simulink model "quadcopter"  (R2023a)
settings: Solver=ode8  StartTime=0.0  StopTime=90  FixedStep=0.009  RelTol=1e-3
InitFcn:
  | addpath(fullfile(pwd, 'data'));  % Add 'data' folder relative to model location
  | run('param.m');
StopFcn:
  | addpath(fullfile(pwd, 'visualizer'));  % Add 'data' folder relative to model location
  | run('InteractiveFlightData.m');
undefined symbols (not defined in the file): attInit, b, d, g, Jm, Jx, Jy, Jz, Kp1H, Kp1Pitch, Kp1Roll, Kp1XY, Kp1Yaw, Kp2H, Kp2Pitch, Kp2Roll, Kp2XY, Kp2Yaw, Kt, Kth, l, m, motorSpinInit, omegaInit, posInit, Ra, u0, U1, velInit
libraries: SignalEditorBlockLib x1
settings Model: Creator=AlterraOnix  LastModifiedBy=AlterraOnix

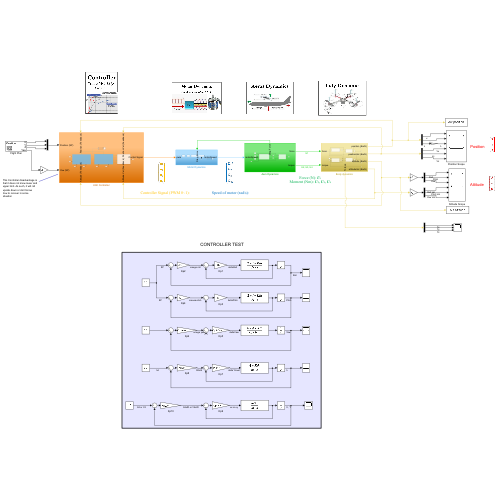
[thumbnail: Simulink's stored preview of the top-level diagram]
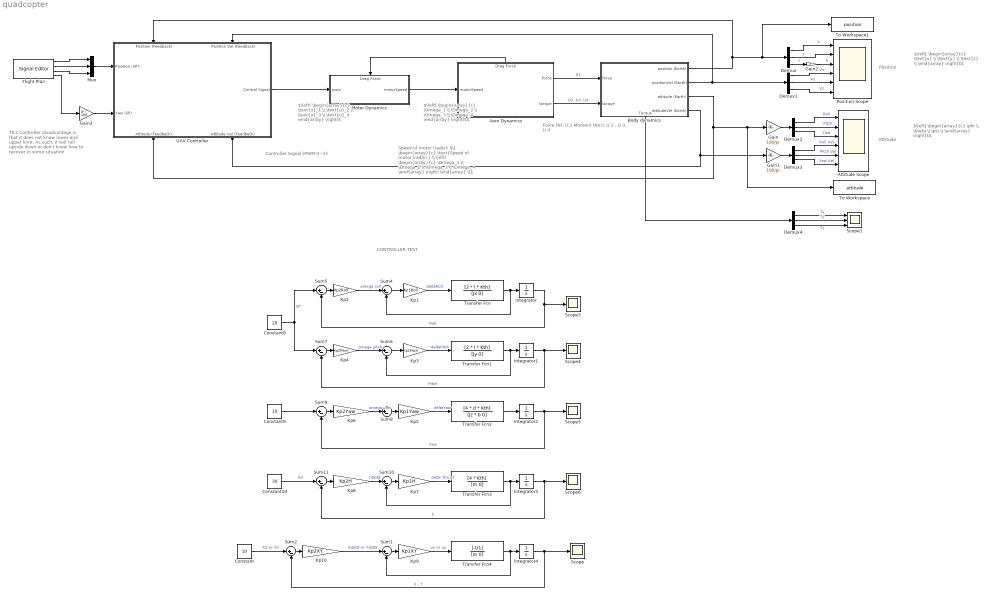
== system quadcopter ==
  note: This Controller disadvantage is that it does not know lower and upper limit. As such, it will roll upside down or don't know how to recover in some situation
  note: Controller Signal (PWM 0~1):
  note: Speed of motor (rad/s): $\[ \begin{array}{c} \text{Speed of motor (rad/s):} \\ \left( \begin{array}{c} \Omega_1 \\ \Omega_2 \\ \Omega_3 \\ \Omega_4 \end{array} \right) \end{array} \]$
  note: CONTROLLER TEST
  note: $\left( \begin{array}{c} \text{u}_1 \\ \text{u}_2 \\ \text{u}_3 \\ \text{u}_4 \end{array} \right)$
  note: $\left( \begin{array}{c} \Omega_1 \\ \Omega_2 \\ \Omega_3 \\ \Omega_4 \end{array} \right)$$
  note: $\left[ \begin{array}{c} \text{x} \\ \text{y} \\ \text{z} \\ \end{array} \right]$$
  note: Attitude
  note: Force (N): U 1
      | Moment (Nm): U 2 , U 3 , U 4
  note: $\left[ \begin{array}{c} \phi \\ \theta \\ \psi \\ \end{array} \right]$$
  note: Position
  Aero Dynamics : Subsystem
      settings: PortSchema="{\"entries\":[{\"content\":{\"sides\":[{\"content\":{\"connectorIds\":[\"In1\"]},\"type\":\"ConnectorPlacement.EquallySpacedRectSide\",\"uuid\":\"5da6d23f-8fa7-4c0d-a7a0-beca667c322f\"},{\"content\":{\"connectorIds\":[\"Out1\",\"Out2\"],\"side\":\"RIGHT\"},\"type\":\"ConnectorPlacement.EquallySpacedRectSide\",\"uuid\":\"114e7ba7-d132-465a-ab12-df00cea923bb\"},{\"content\":{\"connectorIds\":[\"Out3\"],\"side\":\"TOP\"},\"type\":\"ConnectorPlacement.EquallySpacedRectSide\",\"uuid\":\"e5217758-388b-4662-b4f7-0acce50e1924\"},{\"content\":{\"side\":\"BOTTOM\"},\"type\":\"ConnectorPlacement.EquallySpacedRectSide\",\"uuid\":\"6570f914-0b05-4701-b12c-fff372ec49f4\"}]},\"type\":\"ConnectorPlacement.EquallySpacedConnector\",\"uuid\":\"cad8bab3-1cdd-4308-8006-abeb193f8d84\"}],\"packageUris\":[\"http://schema.mathworks.com/mf0/Connector/R2020b\"],\"version\":\"1.0\"}"
  Attitude Scope : Scope  NumInputPorts=6
  Body dynamics : Subsystem
      settings: PortSchema="{\"entries\":[{\"content\":{\"sides\":[{\"content\":{\"connectorIds\":[\"In1\",\"In2\"]},\"type\":\"ConnectorPlacement.EquallySpacedRectSide\",\"uuid\":\"f237c637-46b2-45cc-89c7-502c3b4d3a82\"},{\"content\":{\"connectorIds\":[\"Out1\",\"Out2\",\"Out3\",\"Out4\"],\"side\":\"RIGHT\"},\"type\":\"ConnectorPlacement.EquallySpacedRectSide\",\"uuid\":\"40c9e1e3-93af-41ee-b851-152c56db6279\"},{\"content\":{\"side\":\"TOP\"},\"type\":\"ConnectorPlacement.EquallySpacedRectSide\",\"uuid\":\"88961279-dd7e-4791-8884-b5ffc6cf90cf\"},{\"content\":{\"connectorIds\":[\"Out5\"],\"side\":\"BOTTOM\"},\"type\":\"ConnectorPlacement.EquallySpacedRectSide\",\"uuid\":\"3396dfe3-4d1e-4c48-aaa0-4ba76fac5eff\"}]},\"type\":\"ConnectorPlacement.EquallySpacedConnector\",\"uuid\":\"743c7388-b4e3-439e-b61e-34a6bdced663\"}],\"packageUris\":[\"http://schema.mathworks.com/mf0/Connector/R2020b\"],\"version\":\"1.0\"}"
  Constant : Constant  Value=10
  Constant10 : Constant  Value=30
  Constant8 : Constant  Value=20
  Constant9 : Constant  Value=10
  Demux{,1..4} (5 alike) : Demux  Outputs=3
  Flight Plan : SignalEditorBlockLib/Signal Editor  FileName=flightPlan.mat  ActiveScenario=Position  ActiveSignal=X  IsBus=off  OutputBusObjectStr=Bus: BusObject  SampleTime=0  Interpolate=off  ZeroCross=off  OutputAfterFinalValue=Setting to zero  Unit=inherit  PreserveSignalName=on  ApplySigPropsToAllScenarios=on
  Gain : Gain  Gain=180/pi
  Gain1 : Gain  Gain=180/pi
  Gain2 : Gain  Gain=-1
  Gain3 : Gain  Gain=pi / 180
  Integrator{,1..4} (5 alike) : Integrator
  Kp1 : Gain  Gain=Kp1Roll
  Kp10 : Gain  Gain=Kp2XY
  Kp2 : Gain  Gain=Kp2Roll
  Kp3 : Gain  Gain=Kp1Pitch
  Kp4 : Gain  Gain=Kp2Pitch
  Kp5 : Gain  Gain=Kp1Yaw
  Kp6 : Gain  Gain=Kp2Yaw
  Kp7 : Gain  Gain=Kp1H
  Kp8 : Gain  Gain=Kp2H
  Kp9 : Gain  Gain=Kp1XY
  Motor Dynamics : Subsystem
      settings: PortSchema="{\"entries\":[{\"content\":{\"sides\":[{\"content\":{\"connectorIds\":[\"In1\"]},\"type\":\"ConnectorPlacement.EquallySpacedRectSide\",\"uuid\":\"1ed76e9c-5936-4080-821c-bad0eb24ae59\"},{\"content\":{\"connectorIds\":[\"Out1\"],\"side\":\"RIGHT\"},\"type\":\"ConnectorPlacement.EquallySpacedRectSide\",\"uuid\":\"bcce61fc-9c46-4acb-991d-be4c01e36c5c\"},{\"content\":{\"connectorIds\":[\"In2\"],\"side\":\"TOP\"},\"type\":\"ConnectorPlacement.EquallySpacedRectSide\",\"uuid\":\"b76f1f95-13d4-401e-9c02-e7da8ef90a20\"},{\"content\":{\"side\":\"BOTTOM\"},\"type\":\"ConnectorPlacement.EquallySpacedRectSide\",\"uuid\":\"72a5d901-ef88-4b44-b58a-8f83b182bcfd\"}]},\"type\":\"ConnectorPlacement.EquallySpacedConnector\",\"uuid\":\"e2e8c0d7-4140-446e-9fb7-4366562bc7fa\"}],\"packageUris\":[\"http://schema.mathworks.com/mf0/Connector/R2020b\"],\"version\":\"1.0\"}"
  Mux : Mux  Inputs=3
  Position Scope : Scope  NumInputPorts=6
  Scope{,3..6} (5 alike) : Scope
  Scope1 : Scope  NumInputPorts=3
  Sum{1..2,4..11} (10 alike) : Sum  Inputs=|+-
  To Workspace : ToWorkspace  VariableName=attitude  SaveFormat=Timeseries  SampleTime=-1
  To Workspace1 : ToWorkspace  VariableName=position  SaveFormat=Timeseries  SampleTime=-1
  Transfer Fcn : TransferFcn  Numerator=[2 * l * Kth]  Denominator=[Jx 0]
  Transfer Fcn1 : TransferFcn  Numerator=[2 * l * Kth]  Denominator=[Jy 0]
  Transfer Fcn2 : TransferFcn  Numerator=[4 * d * Kth]  Denominator=[Jz * b 0]
  Transfer Fcn3 : TransferFcn  Numerator=[4 * Kth]  Denominator=[m 0]
  Transfer Fcn4 : TransferFcn  Numerator=[-U1]  Denominator=[m 0]
  UAV Controller : Subsystem
      settings: PortSchema="{\"entries\":[{\"content\":{\"sides\":[{\"content\":{\"connectorIds\":[\"In1\",\"In2\"]},\"type\":\"ConnectorPlacement.EquallySpacedRectSide\",\"uuid\":\"50802edf-a040-4c28-b591-d88e611188de\"},{\"content\":{\"connectorIds\":[\"Out1\"],\"side\":\"RIGHT\"},\"type\":\"ConnectorPlacement.EquallySpacedRectSide\",\"uuid\":\"dce66916-8d71-4fa6-a653-99da5dcfcd3d\"},{\"content\":{\"connectorIds\":[\"In3\",\"In4\"],\"side\":\"TOP\"},\"type\":\"ConnectorPlacement.EquallySpacedRectSide\",\"uuid\":\"d9b7a688-6099-435e-b59a-2f38cb1d0a01\"},{\"content\":{\"connectorIds\":[\"In5\",\"In6\"],\"side\":\"BOTTOM\"},\"type\":\"ConnectorPlacement.EquallySpacedRectSide\",\"uuid\":\"81b63a5f-7537-41dc-8937-f7595f7d4ca8\"}]},\"type\":\"ConnectorPlacement.EquallySpacedConnector\",\"uuid\":\"c3f81b6a-8709-448a-9549-898422283d5d\"}],\"packageUris\":[\"http://schema.mathworks.com/mf0/Connector/R2020b\"],\"version\":\"1.0\"}"
  wires:
  Transfer Fcn/1 -> Sum4/2, Integrator/1
  Kp1/1 -> Transfer Fcn/1  "deltaRoll"
  Sum4/1 -> Kp1/1
  Sum5/1 -> Kp2/1
  Kp2/1 -> Sum4/1  "omega roll"
  Integrator/1 -> Sum5/2, Scope3/1  "Roll"
  Integrator1/1 -> Scope4/1, Sum7/2  "Pitch"
  Sum7/1 -> Kp4/1
  Transfer Fcn1/1 -> Sum6/2, Integrator1/1
  Kp3/1 -> Transfer Fcn1/1  "deltaPitch"
  Sum6/1 -> Kp3/1
  Kp4/1 -> Sum6/1  "omega pitch"
  Kp6/1 -> Sum8/1  "omega yaw"
  Sum8/1 -> Kp5/1
  Integrator2/1 -> Scope5/1, Sum9/2  "Yaw"
  Kp5/1 -> Transfer Fcn2/1  "deltaYaw"
  Constant8/1 -> Sum7/1, Sum5/1  "SP"
  Sum9/1 -> Kp6/1
  Constant9/1 -> Sum9/1
  Transfer Fcn3/1 -> Sum10/2, Integrator3/1
  Integrator3/1 -> Scope6/1, Sum11/2  "h"
  Kp8/1 -> Sum10/1  "hDotd"
  Sum11/1 -> Kp8/1
  Kp7/1 -> Transfer Fcn3/1  "delta' thrust"
  Sum10/1 -> Kp7/1
  Constant10/1 -> Sum11/1  "hd"
  Constant/1 -> Sum2/1  "Xd or Yd"
  Kp9/1 -> Transfer Fcn4/1  "ux or uy"
  Sum2/1 -> Kp10/1
  Kp10/1 -> Sum1/1  "XdotD or YdotD"
  Transfer Fcn4/1 -> Sum1/2, Integrator4/1
  Sum1/1 -> Kp9/1
  Integrator4/1 -> Sum2/2, Scope/1  "X , Y"
  Mux/1 -> UAV Controller/1(Position (SP))
  Demux1/3 -> Position Scope/6  "Vz"
  Demux1/2 -> Position Scope/5  "Vy"
  Demux1/1 -> Position Scope/4  "Vx"
  Demux/2 -> Position Scope/2  "y"
  Demux/1 -> Position Scope/1  "x"
  Gain/1 -> Demux2/1
  Demux2/1 -> Attitude Scope/1  "Roll"
  Demux2/2 -> Attitude Scope/2  "Pitch"
  Demux2/3 -> Attitude Scope/3  "Yaw"
  Gain1/1 -> Demux3/1
  Demux3/1 -> Attitude Scope/4  "Roll Vel"
  Demux3/2 -> Attitude Scope/5  "Pitch Vel"
  Demux3/3 -> Attitude Scope/6  "Yaw Vel"
  Gain2/1 -> Position Scope/3  "h"
  Demux/3 -> Gain2/1  "z"
  UAV Controller/1(Control Signal) -> Motor Dynamics/1(pwm)
  Aero Dynamics/1(force) -> Body dynamics/1(force)  "U1"
  Aero Dynamics/3(Drag Force) -> Motor Dynamics/2(Drag Force)
  Motor Dynamics/1(motorSpeed) -> Aero Dynamics/1(motorSpeed)
  Aero Dynamics/2(torque) -> Body dynamics/2(torque)  "U2, U3, U4"
  Body dynamics/4(attitudeVel (Earth)) -> Gain1/1, UAV Controller/6(Attitude Vel (Feedback))
  Body dynamics/3(attitude (Earth)) -> To Workspace/1, Gain/1, UAV Controller/5(Attitude (Feedback))
  Body dynamics/2(positionVel (Earth)) -> Demux1/1, UAV Controller/4(Position Vel (Feedback))
  Body dynamics/1(position (Earth)) -> UAV Controller/3(Position (Feedback)), To Workspace1/1, Demux/1
  Gain3/1 -> UAV Controller/2(Yaw (SP))
  Body dynamics/5(Torque) -> Demux4/1
  Demux4/3 -> Scope1/3  "Tz"
  Demux4/2 -> Scope1/2  "Ty"
  Demux4/1 -> Scope1/1  "Tx"
  Flight Plan/1 -> Mux/1
  Flight Plan/2 -> Mux/2
  Flight Plan/3 -> Mux/3
  Flight Plan/4 -> Gain3/1
  Transfer Fcn2/1 -> Integrator2/1

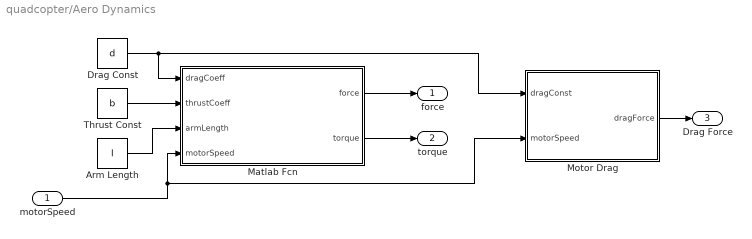
== system quadcopter/Aero Dynamics ==
  motorSpeed : Inport
  Arm Length : Constant  Value=l
  Drag Const : Constant  Value=d
  Matlab Fcn : MATLAB Function  TreatAsAtomicUnit=on
  Motor Drag : MATLAB Function  TreatAsAtomicUnit=on
  Thrust Const : Constant  Value=b
  force : Outport
  torque : Outport  Port=2
  Drag Force : Outport  Port=3
  wires:
  Drag Const/1 -> Motor Drag/1(dragConst), Matlab Fcn/1(dragCoeff)
  Arm Length/1 -> Matlab Fcn/3(armLength)
  Thrust Const/1 -> Matlab Fcn/2(thrustCoeff)
  motorSpeed/1 -> Motor Drag/2(motorSpeed), Matlab Fcn/4(motorSpeed)
  Matlab Fcn/1(force) -> force/1
  Motor Drag/1(dragForce) -> Drag Force/1
  Matlab Fcn/2(torque) -> torque/1

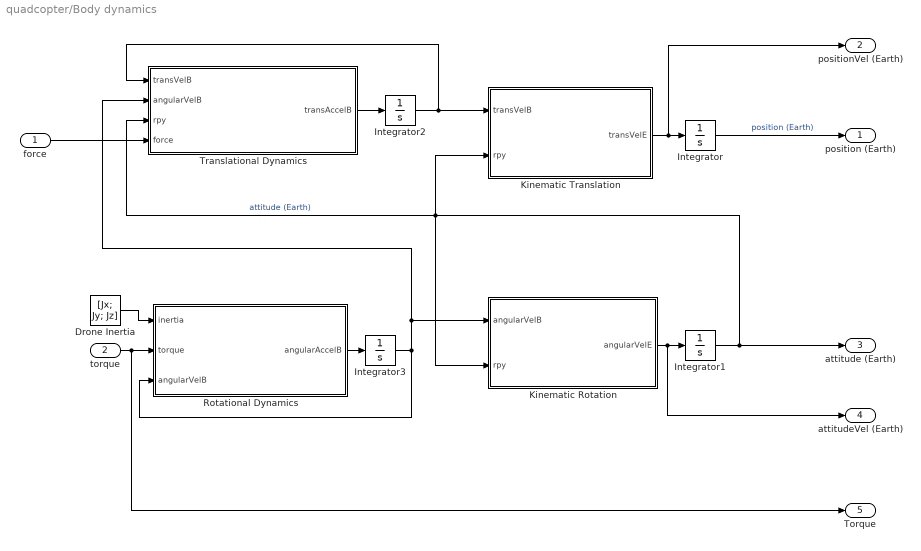
== system quadcopter/Body dynamics ==
  force : Inport
  torque : Inport  Port=2
  Drone Inertia : Constant  Value=[Jx; Jy; Jz]
  Integrator : Integrator  InitialCondition=posInit
  Integrator1 : Integrator  InitialCondition=attInit
  Integrator2 : Integrator  InitialCondition=velInit
  Integrator3 : Integrator  InitialCondition=omegaInit
  Kinematic Rotation : MATLAB Function  TreatAsAtomicUnit=on
  Kinematic Translation : MATLAB Function  TreatAsAtomicUnit=on
  Rotational Dynamics : MATLAB Function  TreatAsAtomicUnit=on
  Translational Dynamics : Subsystem
  position (Earth) : Outport
  positionVel (Earth) : Outport  Port=2
  attitude (Earth) : Outport  Port=3
  attitudeVel (Earth) : Outport  Port=4
  Torque : Outport  Port=5
  wires:
  Kinematic Rotation/1(angularVelE) -> attitudeVel (Earth)/1, Integrator1/1
  Drone Inertia/1 -> Rotational Dynamics/1(inertia)
  Translational Dynamics/1(transAccelB) -> Integrator2/1
  Kinematic Translation/1(transVelE) -> positionVel (Earth)/1, Integrator/1
  Rotational Dynamics/1(angularAccelB) -> Integrator3/1
  Integrator2/1 -> Translational Dynamics/1(transVelB), Kinematic Translation/1(transVelB)
  Integrator1/1 -> Translational Dynamics/3(rpy), Kinematic Rotation/2(rpy), Kinematic Translation/2(rpy), attitude (Earth)/1  "attitude (Earth)"
  Integrator/1 -> position (Earth)/1  "position (Earth)"
  Integrator3/1 -> Rotational Dynamics/3(angularVelB), Translational Dynamics/2(angularVelB), Kinematic Rotation/1(angularVelB)
  torque/1 -> Torque/1, Rotational Dynamics/2(torque)
  force/1 -> Translational Dynamics/4(force)

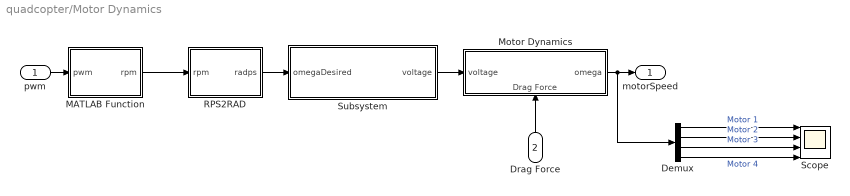
== system quadcopter/Motor Dynamics ==
  pwm : Inport
  Drag Force : Inport  Port=2
  Demux : Demux
  MATLAB Function : MATLAB Function  TreatAsAtomicUnit=on
  Motor Dynamics : Subsystem
      settings: PortSchema="{\"entries\":[{\"content\":{\"sides\":[{\"content\":{\"connectorIds\":[\"In1\"]},\"type\":\"ConnectorPlacement.EquallySpacedRectSide\",\"uuid\":\"c533e7cd-ee38-4db5-be38-3827405b94e5\"},{\"content\":{\"connectorIds\":[\"Out1\"],\"side\":\"RIGHT\"},\"type\":\"ConnectorPlacement.EquallySpacedRectSide\",\"uuid\":\"e10529f3-e7e6-435f-ba64-638186187bc4\"},{\"content\":{\"side\":\"TOP\"},\"type\":\"ConnectorPlacement.EquallySpacedRectSide\",\"uuid\":\"af8a99ba-dd5a-4918-9e60-3f38c4f7af03\"},{\"content\":{\"connectorIds\":[\"In2\"],\"side\":\"BOTTOM\"},\"type\":\"ConnectorPlacement.EquallySpacedRectSide\",\"uuid\":\"cc26d8fe-22a0-44bc-9eba-a7f7a779408e\"}]},\"type\":\"ConnectorPlacement.EquallySpacedConnector\",\"uuid\":\"51d375ef-3caf-4fe1-845a-afb7267c381d\"}],\"packageUris\":[\"http://schema.mathworks.com/mf0/Connector/R2020b\"],\"version\":\"1.0\"}"
  RPS2RAD : MATLAB Function  TreatAsAtomicUnit=on
  Scope : Scope  NumInputPorts=4
  Subsystem : Subsystem
  motorSpeed : Outport
  wires:
  Subsystem/1(voltage) -> Motor Dynamics/1(voltage)
  Motor Dynamics/1(omega) -> Demux/1, motorSpeed/1
  Drag Force/1 -> Motor Dynamics/2(Drag Force)
  MATLAB Function/1(rpm) -> RPS2RAD/1(rpm)
  pwm/1 -> MATLAB Function/1(pwm)
  RPS2RAD/1(radps) -> Subsystem/1(omegaDesired)
  Demux/1 -> Scope/1  "Motor 1"
  Demux/2 -> Scope/2  "Motor 2"
  Demux/3 -> Scope/3  "Motor 3"
  Demux/4 -> Scope/4  "Motor 4"

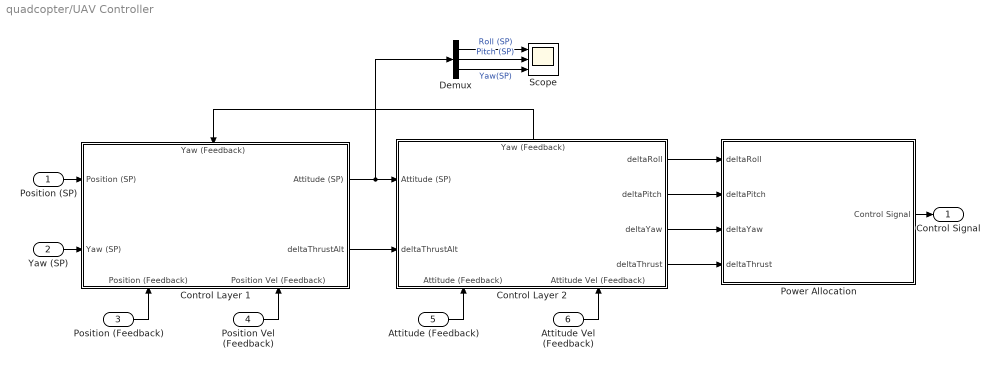
== system quadcopter/UAV Controller ==
  Position (SP) : Inport
  Yaw (SP) : Inport  Port=2
  Position (Feedback) : Inport  Port=3
  Position Vel (Feedback) : Inport  Port=4
  Attitude (Feedback) : Inport  Port=5
  Attitude Vel (Feedback) : Inport  Port=6
  Control Layer 1 : Subsystem
      settings: PortSchema="{\"entries\":[{\"content\":{\"sides\":[{\"content\":{\"connectorIds\":[\"In1\",\"In2\"]},\"type\":\"ConnectorPlacement.EquallySpacedRectSide\",\"uuid\":\"e1a47314-e725-4ad2-912f-1a38871ee891\"},{\"content\":{\"connectorIds\":[\"Out1\",\"Out2\"],\"side\":\"RIGHT\"},\"type\":\"ConnectorPlacement.EquallySpacedRectSide\",\"uuid\":\"53b24631-b87e-42e7-944b-57bbc6991867\"},{\"content\":{\"connectorIds\":[\"In3\"],\"side\":\"TOP\"},\"type\":\"ConnectorPlacement.EquallySpacedRectSide\",\"uuid\":\"7fd7a42b-f6aa-4761-a0eb-10b11e6a4f43\"},{\"content\":{\"connectorIds\":[\"In4\",\"In5\"],\"side\":\"BOTTOM\"},\"type\":\"ConnectorPlacement.EquallySpacedRectSide\",\"uuid\":\"80c3e12e-deab-4463-bb3e-5443ff9a6220\"}]},\"type\":\"ConnectorPlacement.EquallySpacedConnector\",\"uuid\":\"e52dd722-c82f-474b-bf17-6318b1f157b3\"}],\"packageUris\":[\"http://schema.mathworks.com/mf0/Connector/R2020b\"],\"version\":\"1.0\"}"
  Control Layer 2 : Subsystem
      settings: PortSchema="{\"entries\":[{\"content\":{\"sides\":[{\"content\":{\"connectorIds\":[\"In1\",\"In2\"]},\"type\":\"ConnectorPlacement.EquallySpacedRectSide\",\"uuid\":\"ca8a29f1-d2a3-473a-82ed-9fe12abcceea\"},{\"content\":{\"connectorIds\":[\"Out1\",\"Out2\",\"Out3\",\"Out4\"],\"side\":\"RIGHT\"},\"type\":\"ConnectorPlacement.EquallySpacedRectSide\",\"uuid\":\"e4ee1971-4b00-410f-bb76-76195639c31e\"},{\"content\":{\"connectorIds\":[\"Out5\"],\"side\":\"TOP\"},\"type\":\"ConnectorPlacement.EquallySpacedRectSide\",\"uuid\":\"3619c6cc-5c83-4adf-914e-d0bdc3e41505\"},{\"content\":{\"connectorIds\":[\"In3\",\"In4\"],\"side\":\"BOTTOM\"},\"type\":\"ConnectorPlacement.EquallySpacedRectSide\",\"uuid\":\"42efcdc0-00f6-4a08-9fda-d07be9cd5595\"}]},\"type\":\"ConnectorPlacement.EquallySpacedConnector\",\"uuid\":\"bb536f40-a213-48a0-8d9b-f4246912eccc\"}],\"packageUris\":[\"http://schema.mathworks.com/mf0/Connector/R2020b\"],\"version\":\"1.0\"}"
  Demux : Demux  Outputs=3
  Power Allocation : Subsystem
  Scope : Scope  NumInputPorts=3
  Control Signal : Outport
  wires:
  Attitude (Feedback)/1 -> Control Layer 2/3(Attitude (Feedback))
  Control Layer 2/4(deltaThrust) -> Power Allocation/4(deltaThrust)
  Control Layer 2/2(deltaPitch) -> Power Allocation/2(deltaPitch)
  Control Layer 1/1(Attitude (SP)) -> Demux/1, Control Layer 2/1(Attitude (SP))
  Control Layer 2/5(Yaw (Feedback)) -> Control Layer 1/3(Yaw (Feedback))
  Control Layer 2/3(deltaYaw) -> Power Allocation/3(deltaYaw)
  Control Layer 2/1(deltaRoll) -> Power Allocation/1(deltaRoll)
  Control Layer 1/2(deltaThrustAlt) -> Control Layer 2/2(deltaThrustAlt)
  Position (SP)/1 -> Control Layer 1/1(Position (SP))
  Attitude Vel (Feedback)/1 -> Control Layer 2/4(Attitude Vel (Feedback))
  Yaw (SP)/1 -> Control Layer 1/2(Yaw (SP))
  Position (Feedback)/1 -> Control Layer 1/4(Position (Feedback))
  Power Allocation/1(Control Signal) -> Control Signal/1
  Position Vel (Feedback)/1 -> Control Layer 1/5(Position Vel (Feedback))
  Demux/1 -> Scope/1  "Roll (SP)"
  Demux/2 -> Scope/2  "Pitch (SP)"
  Demux/3 -> Scope/3  "Yaw(SP)"

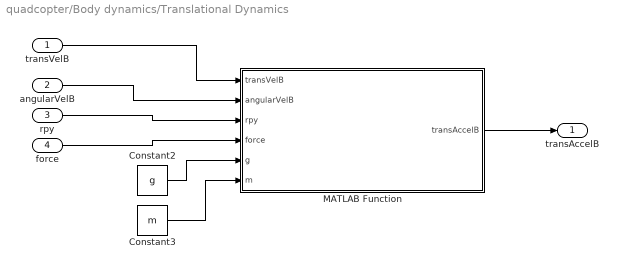
== system quadcopter/Body dynamics/Translational Dynamics ==
  transVelB : Inport
  angularVelB : Inport  Port=2
  rpy : Inport  Port=3
  force : Inport  Port=4
  Constant2 : Constant  Value=g
  Constant3 : Constant  Value=m
  MATLAB Function : MATLAB Function  TreatAsAtomicUnit=on
  transAccelB : Outport
  wires:
  rpy/1 -> MATLAB Function/3(rpy)
  transVelB/1 -> MATLAB Function/1(transVelB)
  Constant2/1 -> MATLAB Function/5(g)
  force/1 -> MATLAB Function/4(force)
  Constant3/1 -> MATLAB Function/6(m)
  angularVelB/1 -> MATLAB Function/2(angularVelB)
  MATLAB Function/1(transAccelB) -> transAccelB/1

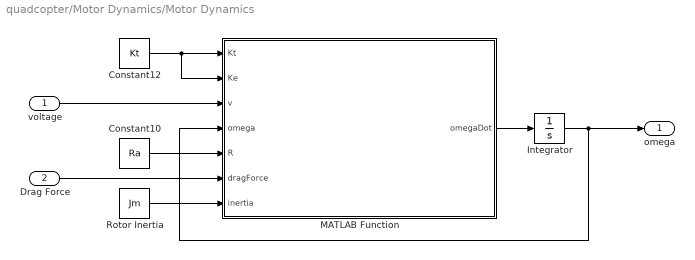
== system quadcopter/Motor Dynamics/Motor Dynamics ==
  voltage : Inport
  Drag Force : Inport  Port=2
  Constant10 : Constant  Value=Ra
  Constant12 : Constant  Value=Kt
  Integrator : Integrator  InitialCondition=motorSpinInit
  MATLAB Function : MATLAB Function  TreatAsAtomicUnit=on
  Rotor Inertia : Constant  Value=Jm
  omega : Outport
  wires:
  Constant12/1 -> MATLAB Function/1(Kt), MATLAB Function/2(Ke)
  voltage/1 -> MATLAB Function/3(v)
  Integrator/1 -> omega/1, MATLAB Function/4(omega)
  MATLAB Function/1(omegaDot) -> Integrator/1
  Constant10/1 -> MATLAB Function/5(R)
  Rotor Inertia/1 -> MATLAB Function/7(inertia)
  Drag Force/1 -> MATLAB Function/6(dragForce)

== system quadcopter/Motor Dynamics/Subsystem ==
  omegaDesired : Inport
  Constant13 : Constant  Value=Ra
  Constant14 : Constant  Value=d
  Constant15 : Constant  Value=Kt
  MATLAB Function : MATLAB Function  TreatAsAtomicUnit=on
  voltage : Outport
  wires:
  Constant13/1 -> MATLAB Function/5(Ra)
  MATLAB Function/1(voltage) -> voltage/1
  omegaDesired/1 -> MATLAB Function/1(omegaDesired)
  Constant15/1 -> MATLAB Function/2(Ke), MATLAB Function/3(Kt)
  Constant14/1 -> MATLAB Function/4(d)

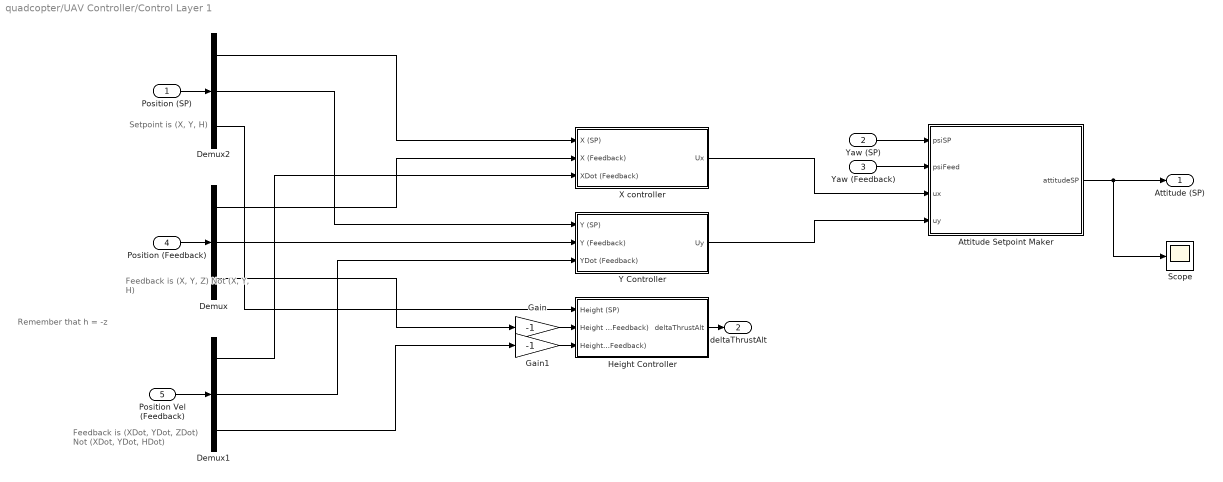
== system quadcopter/UAV Controller/Control Layer 1 ==
  note: Feedback is (X, Y, Z)
      | Not (X, Y, H)
  note: Remember that h = -z
  note: Feedback is (XDot, YDot, ZDot)
      | Not (XDot, YDot, HDot)
  note: Setpoint is (X, Y, H)
  Position (SP) : Inport
  Yaw (SP) : Inport  Port=2
  Yaw (Feedback) : Inport  Port=3
  Position (Feedback) : Inport  Port=4
  Position Vel (Feedback) : Inport  Port=5
  Attitude Setpoint Maker : MATLAB Function  TreatAsAtomicUnit=on
  Demux : Demux  Outputs=3
  Demux1 : Demux  Outputs=3
  Demux2 : Demux  Outputs=3
  Gain : Gain  Gain=-1
  Gain1 : Gain  Gain=-1
  Height Controller : Subsystem
  Scope : Scope
  X controller : Subsystem
  Y Controller : Subsystem
  Attitude (SP) : Outport
  deltaThrustAlt : Outport  Port=2
  wires:
  Height Controller/1(deltaThrustAlt) -> deltaThrustAlt/1
  Position (Feedback)/1 -> Demux/1
  Demux/1 -> X controller/2(X (Feedback))
  Demux/2 -> Y Controller/2(Y (Feedback))
  Gain/1 -> Height Controller/2(Height (Feedback))
  Demux/3 -> Gain/1
  Position Vel (Feedback)/1 -> Demux1/1
  Gain1/1 -> Height Controller/3(HeightDot (Feedback))
  Demux1/3 -> Gain1/1
  Demux1/2 -> Y Controller/3(YDot (Feedback))
  Demux1/1 -> X controller/3(XDot (Feedback))
  Position (SP)/1 -> Demux2/1
  Demux2/1 -> X controller/1(X (SP))
  Demux2/2 -> Y Controller/1(Y (SP))
  Demux2/3 -> Height Controller/1(Height (SP))
  Attitude Setpoint Maker/1(attitudeSP) -> Scope/1, Attitude (SP)/1
  Yaw (SP)/1 -> Attitude Setpoint Maker/1(psiSP)
  X controller/1(Ux) -> Attitude Setpoint Maker/3(ux)
  Y Controller/1(Uy) -> Attitude Setpoint Maker/4(uy)
  Yaw (Feedback)/1 -> Attitude Setpoint Maker/2(psiFeed)

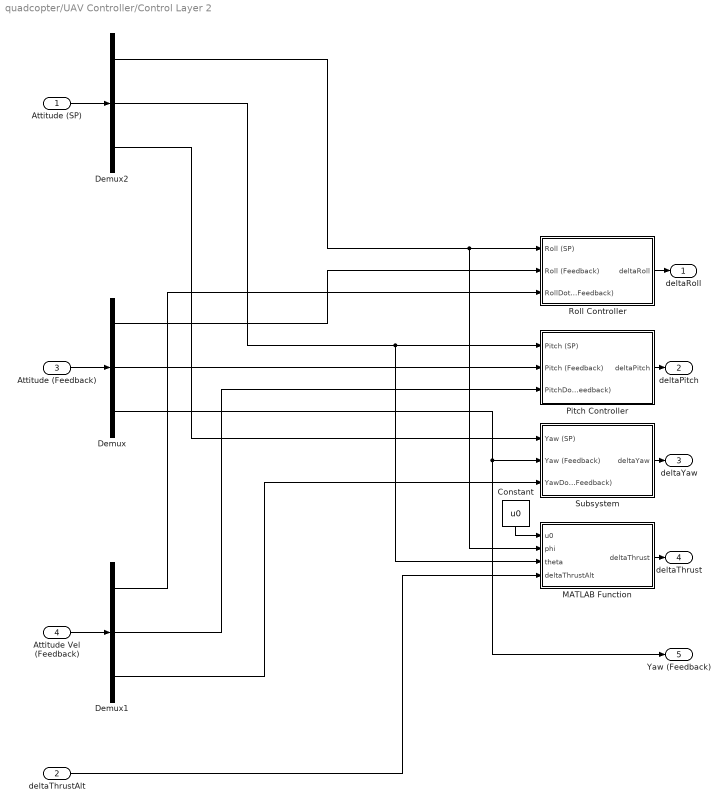
== system quadcopter/UAV Controller/Control Layer 2 ==
  Attitude (SP) : Inport
  deltaThrustAlt : Inport  Port=2
  Attitude (Feedback) : Inport  Port=3
  Attitude Vel (Feedback) : Inport  Port=4
  Constant : Constant  Value=u0
  Demux : Demux  Outputs=3
  Demux1 : Demux  Outputs=3
  Demux2 : Demux  Outputs=3
  MATLAB Function : MATLAB Function  TreatAsAtomicUnit=on
  Pitch Controller : Subsystem
  Roll Controller : Subsystem
  Subsystem : Subsystem
  deltaRoll : Outport
  deltaPitch : Outport  Port=2
  deltaYaw : Outport  Port=3
  deltaThrust : Outport  Port=4
  Yaw (Feedback) : Outport  Port=5
  wires:
  Demux/1 -> Roll Controller/2(Roll (Feedback))
  Roll Controller/1(deltaRoll) -> deltaRoll/1
  Demux1/1 -> Roll Controller/3(RollDot (Feedback))
  Subsystem/1(deltaYaw) -> deltaYaw/1
  Demux/3 -> Yaw (Feedback)/1, Subsystem/2(Yaw (Feedback))
  Demux1/3 -> Subsystem/3(YawDot (Feedback))
  Demux1/2 -> Pitch Controller/3(PitchDot (Feedback))
  Demux/2 -> Pitch Controller/2(Pitch (Feedback))
  Pitch Controller/1(deltaPitch) -> deltaPitch/1
  Attitude (Feedback)/1 -> Demux/1
  Attitude Vel (Feedback)/1 -> Demux1/1
  Attitude (SP)/1 -> Demux2/1
  Demux2/1 -> MATLAB Function/2(phi), Roll Controller/1(Roll (SP))
  Demux2/2 -> MATLAB Function/3(theta), Pitch Controller/1(Pitch (SP))
  Demux2/3 -> Subsystem/1(Yaw (SP))
  deltaThrustAlt/1 -> MATLAB Function/4(deltaThrustAlt)
  MATLAB Function/1(deltaThrust) -> deltaThrust/1
  Constant/1 -> MATLAB Function/1(u0)

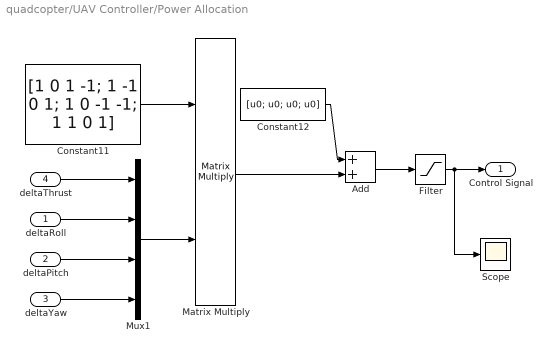
== system quadcopter/UAV Controller/Power Allocation ==
  deltaRoll : Inport
  deltaPitch : Inport  Port=2
  deltaYaw : Inport  Port=3
  deltaThrust : Inport  Port=4
  Add : Sum
  Constant11 : Constant  Value=[1 0 1 -1; 1 -1 0 1; 1 0 -1 -1; 1 1 0 1]
  Constant12 : Constant  Value=[u0; u0; u0; u0]
  Filter : Saturate  UpperLimit=1  LowerLimit=0
  Matrix Multiply : Product  Multiplication=Matrix(*)
  Mux1 : Mux
  Scope : Scope
  Control Signal : Outport
  wires:
  Mux1/1 -> Matrix Multiply/2
  Constant11/1 -> Matrix Multiply/1
  Constant12/1 -> Add/1
  Matrix Multiply/1 -> Add/2
  Filter/1 -> Scope/1, Control Signal/1
  Add/1 -> Filter/1
  deltaPitch/1 -> Mux1/3
  deltaYaw/1 -> Mux1/4
  deltaRoll/1 -> Mux1/2
  deltaThrust/1 -> Mux1/1

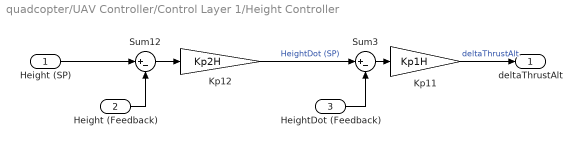
== system quadcopter/UAV Controller/Control Layer 1/Height Controller ==
  Height (SP) : Inport
  Height (Feedback) : Inport  Port=2
  HeightDot (Feedback) : Inport  Port=3
  Kp11 : Gain  Gain=Kp1H
  Kp12 : Gain  Gain=Kp2H
  Sum12 : Sum  Inputs=|+-
  Sum3 : Sum  Inputs=|+-
  deltaThrustAlt : Outport
  wires:
  Kp11/1 -> deltaThrustAlt/1  "deltaThrustAlt"
  Sum3/1 -> Kp11/1
  Sum12/1 -> Kp12/1
  Height (Feedback)/1 -> Sum12/2
  Kp12/1 -> Sum3/1  "HeightDot (SP)"
  Height (SP)/1 -> Sum12/1
  HeightDot (Feedback)/1 -> Sum3/2

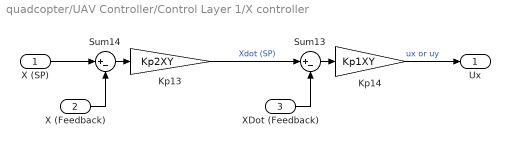
== system quadcopter/UAV Controller/Control Layer 1/X controller ==
  X (SP) : Inport
  X (Feedback) : Inport  Port=2
  XDot (Feedback) : Inport  Port=3
  Kp13 : Gain  Gain=Kp2XY
  Kp14 : Gain  Gain=Kp1XY
  Sum13 : Sum  Inputs=|+-
  Sum14 : Sum  Inputs=|+-
  Ux : Outport
  wires:
  Sum13/1 -> Kp14/1
  Kp14/1 -> Ux/1  "ux or uy"
  X (Feedback)/1 -> Sum14/2
  Kp13/1 -> Sum13/1  "Xdot (SP)"
  Sum14/1 -> Kp13/1
  XDot (Feedback)/1 -> Sum13/2
  X (SP)/1 -> Sum14/1

== system quadcopter/UAV Controller/Control Layer 1/Y Controller ==
  Y (SP) : Inport
  Y (Feedback) : Inport  Port=2
  YDot (Feedback) : Inport  Port=3
  Kp15 : Gain  Gain=Kp2XY
  Kp16 : Gain  Gain=Kp1XY
  Sum15 : Sum  Inputs=|+-
  Sum16 : Sum  Inputs=|+-
  Uy : Outport
  wires:
  Y (SP)/1 -> Sum16/1
  Sum15/1 -> Kp16/1
  Y (Feedback)/1 -> Sum16/2
  Sum16/1 -> Kp15/1
  YDot (Feedback)/1 -> Sum15/2
  Kp16/1 -> Uy/1  "ux or uy"
  Kp15/1 -> Sum15/1  "XdotD or YdotD"

== system quadcopter/UAV Controller/Control Layer 2/Pitch Controller ==
  Pitch (SP) : Inport
  Pitch (Feedback) : Inport  Port=2
  PitchDot (Feedback) : Inport  Port=3
  Kp10 : Gain  Gain=Kp2Pitch
  Kp9 : Gain  Gain=Kp1Pitch
  Sum1 : Sum  Inputs=|+-
  Sum2 : Sum  Inputs=|+-
  deltaPitch : Outport
  wires:
  Pitch (Feedback)/1 -> Sum2/2
  Sum1/1 -> Kp9/1
  Kp10/1 -> Sum1/1  "PitchDot (SP)"
  Kp9/1 -> deltaPitch/1  "deltaPitch"
  Sum2/1 -> Kp10/1
  PitchDot (Feedback)/1 -> Sum1/2
  Pitch (SP)/1 -> Sum2/1

== system quadcopter/UAV Controller/Control Layer 2/Roll Controller ==
  Roll (SP) : Inport
  Roll (Feedback) : Inport  Port=2
  RollDot (Feedback) : Inport  Port=3
  Kp10 : Gain  Gain=Kp2Roll
  Kp9 : Gain  Gain=Kp1Roll
  Sum1 : Sum  Inputs=|+-
  Sum2 : Sum  Inputs=|+-
  deltaRoll : Outport
  wires:
  Kp10/1 -> Sum1/1  "RollDot (SP)"
  Sum2/1 -> Kp10/1
  Roll (SP)/1 -> Sum2/1
  Kp9/1 -> deltaRoll/1  "deltaRoll"
  Roll (Feedback)/1 -> Sum2/2
  Sum1/1 -> Kp9/1
  RollDot (Feedback)/1 -> Sum1/2

== system quadcopter/UAV Controller/Control Layer 2/Subsystem ==
  Yaw (SP) : Inport
  Yaw (Feedback) : Inport  Port=2
  YawDot (Feedback) : Inport  Port=3
  Kp10 : Gain  Gain=Kp2Yaw
  Kp9 : Gain  Gain=Kp1Yaw
  Sum1 : Sum  Inputs=|+-
  Sum2 : Sum  Inputs=|+-
  deltaYaw : Outport
  wires:
  YawDot (Feedback)/1 -> Sum1/2
  Sum2/1 -> Kp10/1
  Kp10/1 -> Sum1/1  "YawDot (SP)"
  Sum1/1 -> Kp9/1
  Yaw (Feedback)/1 -> Sum2/2
  Yaw (SP)/1 -> Sum2/1
  Kp9/1 -> deltaYaw/1  "deltaYaw"

== matlab function quadcopter/Motor Dynamics/RPS2RAD ==
  data: rpm input; radps output
function radps = RPS2RAD(rpm)
    radps = (rpm * 2 * pi) / 60;

== matlab function quadcopter/UAV Controller/Control Layer 2/MATLAB Function ==
  data: u0 input; deltaThrust output; phi input; theta input; deltaThrustAlt input
function deltaThrust = fcn(u0, phi, theta, deltaThrustAlt)
    deltaThrust = ((u0 + deltaThrustAlt) / (cos(phi) * cos(theta))) - u0;

== matlab function quadcopter/UAV Controller/Control Layer 1/Attitude Setpoint Maker ==
  data: psiSP input; psiFeed input; ux input; attitudeSP output; uy input
function attitudeSP = fcn(psiSP, psiFeed, ux, uy)
    
    phiSP_Coeff = ux * sin(psiFeed) - uy * cos(psiFeed);
    phiSP_Coeff = max(min(phiSP_Coeff, 1), -1); % Filter out
    phiSP = asin(phiSP_Coeff);
    phiSP = max(min(phiSP, pi/7), -pi/7);

    thetaSP_Coeff = (ux * cos(psiFeed) + uy * sin(psiFeed)) / cos(phiSP);
    thetaSP_Coeff = max(min(thetaSP_Coeff, 1), -1);
    thetaSP = asin(thetaSP_Coeff);
    thetaSP = max(min(thetaSP, pi/7), -pi/7);
    
    attitudeSP = [phiSP; thetaSP; psiSP];

== matlab function quadcopter/Body dynamics/Kinematic Rotation ==
  data: angularVelB input; angularVelE output; rpy input
function angularVelE = rotationalBE(angularVelB, rpy)
    phi = rpy(1); theta = rpy(2);

    mat = [1            0           -sin(theta);
           0            cos(phi)    sin(phi) * cos(theta);
           0            -sin(phi)   cos(phi) * cos(theta);];

    angularVelE = inv(mat) * angularVelB;

== matlab function quadcopter/Body dynamics/Kinematic Translation ==
  data: transVelB input; transVelE output; rpy input
function transVelE = translationBE(transVelB, rpy)
    phi = rpy(1);
    theta = rpy(2);
    psi = rpy(3);

    rollMat = [1   0   0;
            0   cos(phi)    sin(phi);
            0   -sin(phi)   cos(phi);];

    pitchMat = [cos(theta)  0   -sin(theta);
                0           1   0;
                sin(theta)  0   cos(theta);];

    yawMat = [cos(psi)  sin(psi)    0;
              -sin(psi) cos(psi)    0;
              0         0           1;];

    rotMat = rollMat * pitchMat * yawMat;
    R = [cos(theta)*cos(psi) cos(psi)*sin(theta)*sin(phi) - cos(phi)*sin(psi)  sin(phi)*sin(psi) + cos(phi)*cos(psi)*sin(theta);
        cos(theta)*sin(psi) cos(phi)*cos(psi) + sin(theta)*sin(phi)*sin(psi)  cos(phi)*sin(theta)*sin(psi) - cos(psi)*sin(phi);
        -sin(theta)                               cos(theta)*sin(phi)                               cos(theta)*cos(phi)];

    transVelE = inv(rotMat) * transVelB;

== matlab function quadcopter/Body dynamics/Translational Dynamics/MATLAB Function ==
  data: transAccelB output; transVelB input; angularVelB input; rpy input; force input; g input; m input
function transAccelB = fcn(transVelB, angularVelB, rpy, force, g, m)
    phi = rpy(1); theta = rpy(2);
    rotatateGrav = [-g * sin(theta); 
                    g * sin(phi) * cos(theta); 
                    g * cos(phi) * cos(theta);];
    
    transAccelB = rotatateGrav + (1 / m) * [0; 0; -force] - cross(angularVelB, transVelB);

== matlab function quadcopter/Body dynamics/Rotational Dynamics ==
  data: inertia input; angularAccelB output; torque input; angularVelB input
function angularAccelB = fcn(inertia, torque, angularVelB)
    Jmatrix = diag(inertia);
    angularAccelB = inv(Jmatrix) * (torque - cross(angularVelB, inertia .* angularVelB));

== matlab function quadcopter/Aero Dynamics/Matlab Fcn ==
  data: force output; dragCoeff input; torque output; thrustCoeff input; armLength input; motorSpeed input
function [force, torque] = fcn(dragCoeff, thrustCoeff, armLength, motorSpeed)
    b = thrustCoeff;
    d = dragCoeff;
    l = armLength;

    transformMat = [b       b       b       b;
                    0       -l*b    0       l*b;
                    l*b     0       -l*b    0;
                    -d      d       -d      d;];
    dynamics = transformMat * (motorSpeed .* motorSpeed);
    for i = 1: 4
        if abs(dynamics(i)) < 1e-5
            dynamics(i) = 0;
        end
    end
    force = dynamics(1);
    torque = dynamics(2:4);

== matlab function quadcopter/Motor Dynamics/Motor Dynamics/MATLAB Function ==
  data: Kt input; omegaDot output; Ke input; v input; omega input; R input; dragForce input; inertia input
function omegaDot = fcn(Kt, Ke, v, omega, R, dragForce, inertia)
    omegaDot = (Kt * (v - omega * Ke) / R - dragForce) / inertia;

== matlab function quadcopter/Motor Dynamics/Subsystem/MATLAB Function ==
  data: omegaDesired input; voltage output; Ke input; Kt input; d input; Ra input
function voltage = fcn(omegaDesired, Ke, Kt, d, Ra)
    voltage = Ke * omegaDesired + d * (omegaDesired .^ 2) * Ra / Kt;

== matlab function quadcopter/Motor Dynamics/MATLAB Function ==
  data: pwm input; rpm output
function rpm = PWM2RPM(pwm)
    rpm = 1075 + 7525 * pwm; % Based signal + signal range * strength

== matlab function quadcopter/Aero Dynamics/Motor Drag ==
  data: dragConst input; dragForce output; motorSpeed input
function dragForce = fcn(dragConst, motorSpeed)
    dragForce = dragConst * (motorSpeed .^ 2);
